simulink model "mtrmodel"  (R2020b)
settings: Solver=VariableStepAuto  StartTime=0.0  StopTime=3  RelTol=1e-3
values from neighbouring files (symbols this model uses):
  Ki = (kv*T)/gz    [PID Katsayilari.m]
undefined symbols (not defined in the file or in its folder): B, J, Kb, La, Ra
settings Model: Creator=HCS  LastModifiedBy=HCS

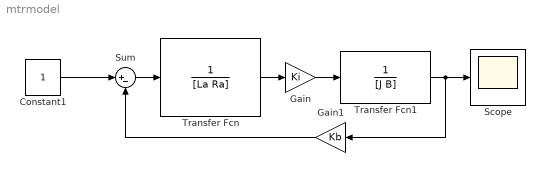
== system mtrmodel ==
  Constant1 : Constant
  Gain : Gain  Gain=Ki
  Gain1 : Gain  Gain=Kb
  Scope : Scope
  Sum : Sum  Inputs=|+-
  Transfer Fcn : TransferFcn  Denominator=[La Ra]
  Transfer Fcn1 : TransferFcn  Denominator=[J B]
  wires:
  Gain/1 -> Transfer Fcn1/1
  Transfer Fcn1/1 -> Scope/1, Gain1/1
  Transfer Fcn/1 -> Gain/1
  Gain1/1 -> Sum/2
  Sum/1 -> Transfer Fcn/1
  Constant1/1 -> Sum/1
